simulink model "DC_Motor_Closed_loop_HystressisPWM"  (R2021a)
settings: Solver=VariableStepAuto  StartTime=0.0  StopTime=1  RelTol=1e-3
InitFcn:
  | Kf=.1;
  | 
  | Ra=2;
  | La=5.2*10^(-3);
  | 
  | j=1.5e-4;
  | B=1e-3;
  | 
  | Imin=0;
  | Imax=20;
libraries: pid_lib x1
settings Model: Creator=User  LastModifiedBy=User
settings SolverCC: AlgebraicLoopSolver=TrustRegion
settings DebuggingCC: SFMachineParentedDataDiag=warning

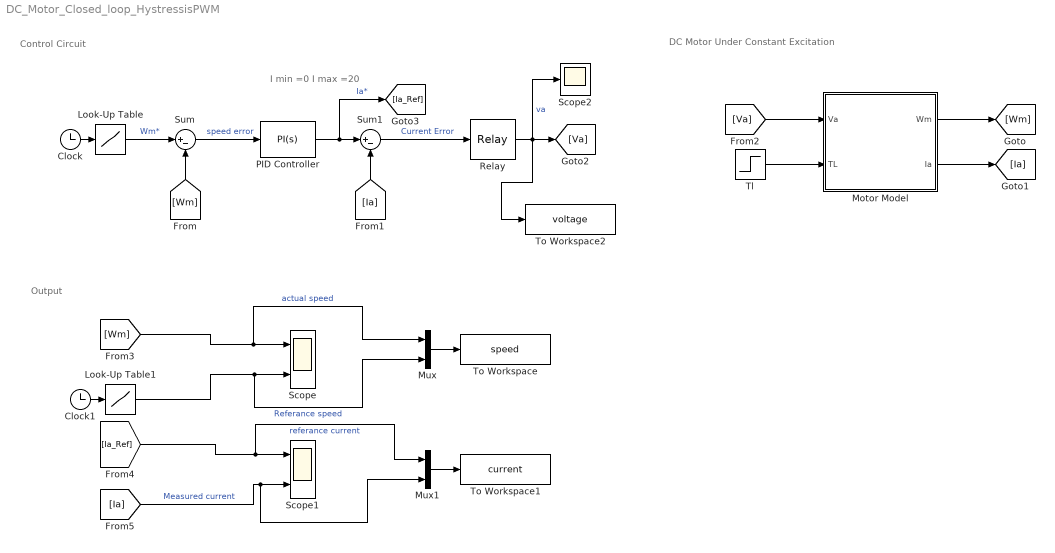
== system DC_Motor_Closed_loop_HystressisPWM ==
  note: Output
  note: Control Circuit
  note: I min =0
      | I max =20
  note: DC Motor Under Constant Excitation
  Clock : Clock
  Clock1 : Clock
  Look-Up Table : Lookup  InputValues=[0 .03 .03 .08 0.1 0.5 0.6 0.8]  Table=[100 100 50 50 100 100 300 300]  SaturateOnIntegerOverflow=on
  Look-Up Table1 : Lookup  InputValues=[0 .03 .03 .08 0.1 0.5 0.6 0.8]  Table=[100 100 50 50 100 100 300 300]  SaturateOnIntegerOverflow=on
  Motor Model : Subsystem
  Mux : Mux  Inputs=2
  Mux1 : Mux  Inputs=2
  PID Controller : pid_lib/PID Controller  Controller=PI  Form=Parallel  TimeDomain=Continuous-time  UseExternalTs=off  SampleTime=-1  IntegratorMethod=Forward Euler  FilterMethod=Forward Euler  ControllerParametersSource=internal  P=1.5  I=100  D=0  UseFilter=on  N=100  TunerSelectOption=Transfer Function Based (PID Tuner App)  InitialConditionSource=internal  InitialConditionForIntegrator=0  InitialConditionForFilter=0  DifferentiatorICPrevScaledInput=0  ExternalReset=none  TrackingMode=off  Kt=1  LimitOutput=on  SatLimitsSource=internal  UpperSaturationLimit=Imax  LowerSaturationLimit=Imin  LinearizeAsGain=on  AntiWindupMode=none  Kb=1  POutMin=[]  POutMax=[]  IOutMin=[]  IOutMax=[]  DOutMin=[]  DOutMax=[]  NOutMin=[]  NOutMax=[]  SumOutMin=[]  SumOutMax=[]  SaturationOutMin=[]  SaturationOutMax=[]  PParamMin=[]  PParamMax=[]  IParamMin=[]  IParamMax=[]  DParamMin=[]  DParamMax=[]  NParamMin=[]  NParamMax=[]  KbParamMin=[]  KbParamMax=[]  KtParamMin=[]  KtParamMax=[]  KbOutMin=[]  KbOutMax=[]  KtOutMin=[]  KtOutMax=[]  IntegratorOutMin=[]  IntegratorOutMax=[]  FilterOutMin=[]  FilterOutMax=[]  SumI1OutMin=[]  SumI1OutMax=[]  SumI2OutMin=[]  SumI2OutMax=[]  SumI3OutMin=[]  SumI3OutMax=[]  SumI4OutMin=[]  SumI4OutMax=[]  SumDOutMin=[]  SumDOutMax=[]  DifferentiatorOutMin=[]  DifferentiatorOutMax=[]  FilterDiffOutCoefMin=[]  FilterDiffOutCoefMax=[]  ReciprocalOutMin=[]  ReciprocalOutMax=[]  SumDenOutMin=[]  SumDenOutMax=[]  SumNumOutMin=[]  SumNumOutMax=[]  DivideOutMin=[]  DivideOutMax=[]  UdiffTsProdOutMin=[]  UdiffTsProdOutMax=[]  NTsProdOutMin=[]  NTsProdOutMax=[]  UintegralTsProdOutMin=[]  UintegralTsProdOutMax=[]  UngainTsProdOutMin=[]  UngainTsProdOutMax=[]  IntegratorContinuousStateAttributes=''  IntegratorStateMustResolveToSignalObject=off  IntegratorRTWStateStorageClass=Auto  FilterContinuousStateAttributes=''  FilterStateMustResolveToSignalObject=off  FilterRTWStateStorageClass=Auto  ParallelPVariant=InternalParameters  IdealPVariant=Disabled  IVariant=InternalParameters  DVariant=Disabled  IntegratorVariant=Continuous  SatVariant=Enabled  AWVariant=Passthrough  PCopyVariant=Disabled  TRVariant=Disabled  FdbkBlocksVariant=Forward  IdealPFdbkVariant=Disabled  SatFdbkVariant=Disabled  DerivativeFilterVariant=Disabled  NVariant=Disabled  NCopyVariant=Disabled_SignalSpec  FilterICVariant=Disabled  IntegratorICVariant=InternalICs  ExternalResetVariant=Disabled  TRSumVariant=Passthrough  SumFdbkVariant=Disabled  SumVariant=Sum_PI  TsampFilterVariant=InternalTs  TsampNgainVariant=Passthrough  TsampIntegralVariant=Passthrough  ExternalSaturationOutDataTypeStr=Inherit: Same as second input
  Relay : Relay  OnSwitchValue=2  OffSwitchValue=-2  OnOutputValue=60
  Scope : Scope  NumInputPorts=2
  Scope1 : Scope  NumInputPorts=2
  Scope2 : Scope
  Sum : Sum  Inputs=|+-
  Sum1 : Sum  Inputs=|+-
  Tl : Step  Time=0.5  Before=1  SampleTime=0
  To Workspace : ToWorkspace  VariableName=speed  SaveFormat=Timeseries  SampleTime=-1
  To Workspace1 : ToWorkspace  VariableName=current  SaveFormat=Timeseries  SampleTime=-1
  To Workspace2 : ToWorkspace  VariableName=voltage  SaveFormat=Timeseries  SampleTime=-1
  wires:
  Look-Up Table/1 -> Sum/1  "Wm*"
  [Wm] -> Sum/2
  Sum/1 -> PID Controller/1  "speed error"
  PID Controller/1 -> [Ia_Ref], Sum1/1  "Ia*"
  [Ia] -> Sum1/2
  Sum1/1 -> Relay/1  "Current Error"
  Clock/1 -> Look-Up Table/1
  Relay/1 -> Scope2/1, [Va], To Workspace2/1  "va"
  Motor Model/1(Wm) -> [Wm]
  Tl/1 -> Motor Model/2(TL)
  Motor Model/2(Ia) -> [Ia]
  [Va] -> Motor Model/1(Va)
  [Wm] -> Mux/1, Scope/1  "actual speed"
  Clock1/1 -> Look-Up Table1/1
  Look-Up Table1/1 -> Mux/2, Scope/2  "Referance speed"
  [Ia_Ref] -> Mux1/1, Scope1/1  "referance current"
  [Ia] -> Mux1/2, Scope1/2  "Measured current"
  Mux/1 -> To Workspace/1
  Mux1/1 -> To Workspace1/1

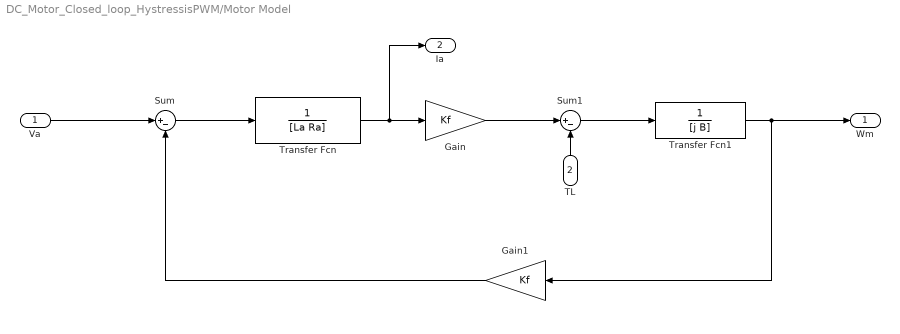
== system DC_Motor_Closed_loop_HystressisPWM/Motor Model ==
  Va : Inport
  TL : Inport  Port=2
  Gain : Gain  Gain=Kf
  Gain1 : Gain  Gain=Kf
  Sum : Sum  Inputs=|+-
  Sum1 : Sum  Inputs=|+-
  Transfer Fcn : TransferFcn  Denominator=[La Ra]
  Transfer Fcn1 : TransferFcn  Denominator=[j B]
  Wm : Outport
  Ia : Outport  Port=2
  wires:
  Gain1/1 -> Sum/2
  Sum/1 -> Transfer Fcn/1
  Transfer Fcn1/1 -> Wm/1, Gain1/1
  TL/1 -> Sum1/2
  Transfer Fcn/1 -> Ia/1, Gain/1
  Sum1/1 -> Transfer Fcn1/1
  Gain/1 -> Sum1/1
  Va/1 -> Sum/1
